simulink model "S_PIL_PVSISTEM_2026_V1"  (R2017a)
settings: Solver=VariableStepAuto  StartTime=0.0  StopTime=1.3  FixedStep=1e-6  MaxStep=1e-4  RelTol=1e-3
values from neighbouring files (symbols this model uses):
  a = 9    [M_PARAM_V1.m]    (also in M_PIL_PVSISTEM_2026_V1.m; ModTusk_V1.m)
  Alpha1 = 2*Zeta_obs*wn_obs    (= 2)    [M_PARAM_V1.m]    (also in M_PIL_PVSISTEM_2026_V1.m)
  Alpha2 = wn_obs    (= 1)    [M_PARAM_V1.m]    (also in M_PIL_PVSISTEM_2026_V1.m)
  alpha_max = 4/ts_min    (= 13333.3333333)    [M_PARAM_V1.m]    (also in M_PIL_PVSISTEM_2026_V1.m; ModTusk_V1.m)
  alpha_min = 4/ts_max    (= 259.067357513)    [M_PARAM_V1.m]    (also in M_PIL_PVSISTEM_2026_V1.m = 133.333333333; ModTusk_V1.m = 133.333333333)
  Cdc = Cdc    (= 0.0033)    [M_PARAM_V1.m]    (also in M_PIL_PVSISTEM_2026_V1.m = 0.00047)
  Cpv = Cpv    (= 0.0001)    [M_PARAM_V1.m]    (also in M_PIL_PVSISTEM_2026_V1.m = 0.0002)
  dIL = (vpv/L)*d*Ts    (= 0.46035072)    [M_PIL_PVSISTEM_2026_V1.m]
  Epsilon = Ep_cont/Ts1    [M_PARAM_V1.m]    (also in M_PIL_PVSISTEM_2026_V1.m)
  ESRCdc = ESRCdc    (= 0.2)    [M_PARAM_V1.m]    (also in M_PIL_PVSISTEM_2026_V1.m)
  ESRCpv = ESRCpv    (= 0.2)    [M_PARAM_V1.m]    (also in M_PIL_PVSISTEM_2026_V1.m)
  Fred = fs    (= 60)    [M_PARAM_V1.m]    (also in M_PIL_PVSISTEM_2026_V1.m)
  fs = 60    [M_PARAM_V1.m]    (also in M_PIL_PVSISTEM_2026_V1.m)
  Icc_calc = In/(5/100)    [M_PARAM_V1.m]    (also in M_PIL_PVSISTEM_2026_V1.m)
  K1 = Kt_acker_d    [M_PARAM_V1.m]    (also in M_PIL_PVSISTEM_2026_V1.m)
  K1y2md = Kmd(1:end-1)    [M_PARAM_V1.m]    (also in M_PIL_PVSISTEM_2026_V1.m)
  Kdpwm = 1/Ucmax    (= 0.000111111111111)    [M_PARAM_V1.m]    (also in M_PIL_PVSISTEM_2026_V1.m = 1.52590218967e-05)
  KI1 = Kp1/Ti1*Ts1    (= 760)    [M_PARAM_V1.m]    (also in M_PIL_PVSISTEM_2026_V1.m = 14.4)
  KI2 = Ki2*Ts4    [M_PARAM_V1.m]    (also in M_PIL_PVSISTEM_2026_V1.m)
  KI4 = Ki4*Ts4    [M_PARAM_V1.m]    (also in M_PIL_PVSISTEM_2026_V1.m)
  KI5 = Ki5*Ts_inv    (= 0.17765287922)    [M_PARAM_V1.m]    (also in M_PIL_PVSISTEM_2026_V1.m = 0.0710611516878)
  Kimd = -Kmd(end)    [M_PARAM_V1.m]    (also in M_PIL_PVSISTEM_2026_V1.m)
  KP1 = Kp1-KI1/2    (= 5320)    [M_PARAM_V1.m]    (also in M_PIL_PVSISTEM_2026_V1.m = 2392.8)
  KP2 = Kp2-KI2/2    [M_PARAM_V1.m]    (also in M_PIL_PVSISTEM_2026_V1.m)
  KP4 = Kp4-KI4/2    [M_PARAM_V1.m]    (also in M_PIL_PVSISTEM_2026_V1.m)
  KP5 = Kp5*Ts_inv-KI5/2    (= -0.0874937760062)    [M_PARAM_V1.m]    (also in M_PIL_PVSISTEM_2026_V1.m = -0.0349975104025)
  L = L    (= 0.0044)    [M_PARAM_V1.m]    (also in M_PIL_PVSISTEM_2026_V1.m = 0.1)
  Linv = 0.03    [M_PARAM_V1.m]    (also in M_PIL_PVSISTEM_2026_V1.m = 0.035)
  Rinv = 0.0417    [M_PARAM_V1.m]    (also in M_PIL_PVSISTEM_2026_V1.m)
  RL = RL    (= 0.494)    [M_PARAM_V1.m]    (also in M_PIL_PVSISTEM_2026_V1.m = 0.3)
  S = 10e3*3/2    (= 15000)    [M_PARAM_V1.m]    (also in M_PIL_PVSISTEM_2026_V1.m)
  Ts = Ts1    (= 0.0002)    [M_PARAM_V1.m]    (also in M_PIL_PVSISTEM_2026_V1.m)
  Ts1 = 1/Fs    (= 0.0002)    [M_PARAM_V1.m]    (also in M_PIL_PVSISTEM_2026_V1.m)
  Ts4 = 1/(4*Fc)    (= 0.000125)    [M_PARAM_V1.m]    (also in M_PIL_PVSISTEM_2026_V1.m = 5e-05)
  Ts_inv = 1/(100*Fc)    (= 5e-06)    [M_PARAM_V1.m]    (also in M_PIL_PVSISTEM_2026_V1.m = 2e-06)
  Ucmax = 9000    [M_PARAM_V1.m]    (also in M_PIL_PVSISTEM_2026_V1.m = 65535)
  vdc = 12    [M_PARAM_V1.m]    (also in M_PIL_PVSISTEM_2026_V1.m = 1000)
  vdc_ref = vdc    (= 12)    [M_PARAM_V1.m]    (also in M_PIL_PVSISTEM_2026_V1.m = 1000)
  Vf = VL/sqrt(3)    [M_PARAM_V1.m]    (also in M_PIL_PVSISTEM_2026_V1.m)
  VL = (381.051/2)    (= 190.5255)    [M_PARAM_V1.m]    (also in M_PIL_PVSISTEM_2026_V1.m)
undefined symbols (not defined in the file or in its folder): DiscIntNeverNeededParam
undefined symbols (not defined in the file): Fs
libraries: powerlib x15, powerlib_meascontrol x12, dsparch4 x3, re_lib x1
(part 1 of 2)
settings Model: ExtModeTrigDuration=10  Creator=dricl  LastModifiedBy=dricl
settings SolverCC: MaxConsecutiveZCs=100000
settings OptimizationCC: PassReuseOutputArgsAs=Individual arguments  MaxStackSize=2560
settings DebuggingCC: ParameterTunabilityLossMsg=error
settings HardwareCC: ProdBitPerPointer=32  ProdBitPerSizeT=32  ProdBitPerPtrDiffT=32  ProdLargestAtomicInteger=Long  ProdLargestAtomicFloat=Double  ProdWordSize=32  ProdLongLongMode=on  ProdHWDeviceType=ARM Compatible->ARM Cortex
settings SFSimCC: MATLABDynamicMemAlloc=off
settings RTWCC: SystemTargetFile=ert.tlc  HardwareBoard=TI Concerto F28M35x (ARM Cortex-M3)  TLCOptions=-aInlineSetEventsForThisBaseRateFcn=TLC_FALSE -aSuppressMultiTaskScheduler=TLC_FALSE -aRateBasedStepFcn=1  TemplateMakefile=ert_default_tmf  Description=Embedded Coder  GenerateReport=on  Toolchain=Texas Instruments Code Composer Studio v6 (ARM)  IncludeHyperlinkInReport=on  LaunchReport=on  CreateSILPILBlock=PIL  GenerateTraceInfo=on  GenerateTraceReport=on  GenerateTraceReportSl=on  GenerateTraceReportSf=on  GenerateTraceReportEml=on
settings CodeAppCC: ForceParamTrailComments=on  IgnoreCustomStorageClasses=off  OperatorAnnotations=on  SimulinkDataObjDesc=on  SFDataObjDesc=on  MATLABFcnDesc=on  InsertBlockDesc=on  MATLABSourceComments=on
settings ERTTargetCC: SupportVariableSizeSignals=on

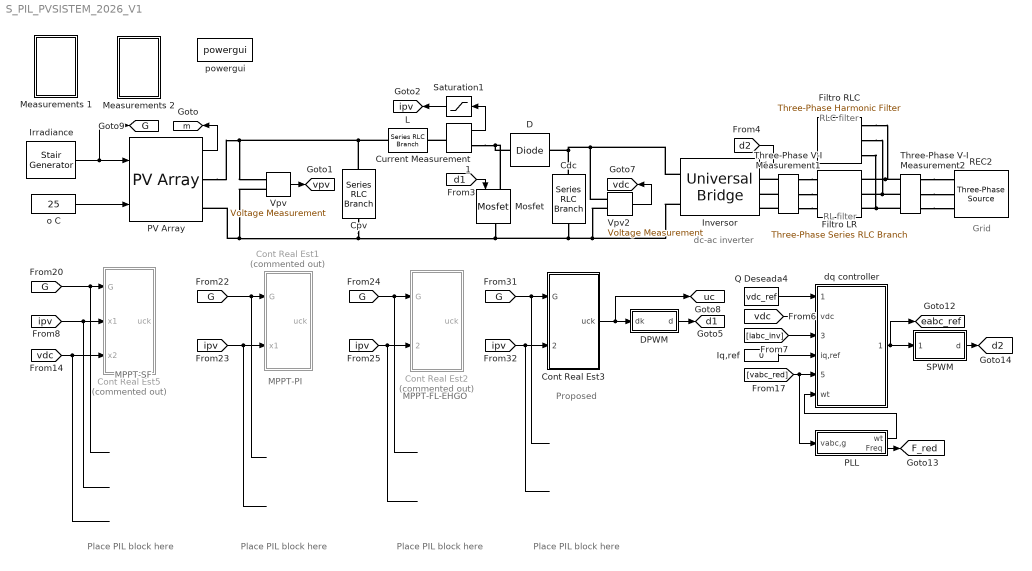
== system S_PIL_PVSISTEM_2026_V1 ==
  note: Place PIL block here
  note: Grid
  note: RLC filter
  note: MPPT-SF
  note: MPPT-PI
  note: MPPT-FL-EHGO
  note: RL filter
  note: dc-ac inverter
  note: Proposed
  note: Place PIL block here
  note: Place PIL block here
  note: Place PIL block here
  Cdc : powerlib/Elements/Series RLC Branch  LConnTagsString=__new0  RConnTagsString=__new0  BranchType=C  Resistance=ESRCdc  Inductance=1e-3  SetiL0=off  InitialCurrent=0  Capacitance=Cdc  Setx0=on  InitialVoltage=vdc_ref  Measurements=None
  Cont Real Est1 : Subsystem  Priority=7  Commented=on
  Cont Real Est2 : Subsystem  Priority=7  Commented=on
  Cont Real Est3 : Subsystem  Priority=7
  Cont Real Est5 : Subsystem  Priority=9  Commented=on
  Cpv : powerlib/Elements/Series RLC Branch  LConnTagsString=__new0  RConnTagsString=__new0  BranchType=C  Resistance=ESRCpv  Inductance=1e-3  SetiL0=off  InitialCurrent=0  Capacitance=Cpv  Setx0=on  InitialVoltage=640.8  Measurements=None
  Current Measurement1 : powerlib/Measurements/Current Measurement  PhasorSimulation=off  OutputType=Complex  PSBequivalent=0
  D : powerlib/Power Electronics/Diode  Ron=Rondiode  Lon=0  Vf=Vfdiode  IC=0  UseSnubber=0  Rs=500  Cs=250e-9  Measurements=off
  DPWM : Subsystem  AncestorBlock=plecslib_extras2/Modulators/Symmetrical PWM  mask(Symmetrical PWM){sampling=Natural (carrier starts with 0), fc=Fs, offset=0, input_limits=[0 Ucmax], output_values=[0 1]}
      mask prompts: fc "Carrier frequency (Hz):"; offset "Carrier offset (p.u.):"; input_limits "Input limits [min max]:"; output_values "Output values [off on]:"
      mask help: PWM generator with a symmetrical triangular carrier. If the input is a vector, the output is also a vector of the same width.
      mask init:
      | if numel(fc)>1 || fc<=0,
      |   error('Carrier frequency must be a positive scalar.');
      | end
      | if numel(offset)>1 || offset<0 || offset>=1,
      |   error('Carrier offset must be a scalar in the range [0; 1/fc[.');
      | end
      | if sampling == 1,
      |   offset = mod(offset+.75, 1);
      | end
      | 
      | si = [.5 mod(offset, .5)]/fc;
      mask Help: eval('plecs(''help'', ''symmetricalpwm.html'')')
      mask TypeOptions sampling: Natural (carrier starts with 0) | Natural (carrier starts with 1) | Regular (double edge) | Regular (single edge)
  Filtro LR : powerlib/Elements/Three-Phase Series RLC Branch  LConnTagsString=A|B|C  RConnTagsString=A|B|C  BranchType=RL  Resistance=Rinv  Inductance=Linv  Capacitance=1e-6  Measurements=None
  Filtro RLC : powerlib/Elements/Three-Phase Harmonic Filter  LConnTagsString=A|B|C  FilterType=Single-tuned  FilterConnection=Y (grounded)  ParNom=[VL fs]  Qc=S*0.001  Fr=[31.42*60]  Frd=[40*fs 80*fs]  Q=5  Measurements=None
      settings: AttributesFormatString=\n  SourceProductName=Simscape Power Systems  SourceProductBaseCode=PS
  Inversor : powerlib/Power Electronics/Universal Bridge  Arms=3  SnubberResistance=1e5  SnubberCapacitance=inf  Device=IGBT / Diodes  Ron=1e-3  Lon=0  ForwardVoltages="[  0  0  ]"  ForwardVoltage=0  GTOparameters=[ 10e-6 , 20e-6 ]  IGBTparameters=[ 1e-6 , 2e-6 ]  Measurements=None  Measurements_2=None  converterType=Rectifier
  Iq,ref : Constant  Value=0  SampleTime=Ts4
  Irradiance : powerlib_meascontrol/Pulse & Signal Generators/Stair Generator  t=[0, 0.1, 0.3, 0.5, 0.7, 0.9, 1.1]  e=[0, 1000, 400, 800, 500, 900, 600]  Ts=0
      settings: SourceProductName=Simscape Power Systems
  L : powerlib/Elements/Series RLC Branch  LConnTagsString=__new0  RConnTagsString=__new0  BranchType=L  Resistance=RL  Inductance=L  SetiL0=off  InitialCurrent=0  Capacitance=1e-6  Setx0=off  InitialVoltage=0  Measurements=None
  Measurements 1 : Subsystem
  Measurements 2 : Subsystem
  Mosfet : powerlib/Power Electronics/Mosfet  Ron=Ronfet  Lon=0  Rd=0  Vfd=0  IC=0  Rs=1e5  Cs=inf  Measurements=off
  PLL : Subsystem
  PV Array : re_lib/Solar/PV Array  Npar=No_Cadenas_Paralelo  Nser=No_Modulos_PorCadena  PlotType=array @ 25 deg.C & specified irradiances  S_vec=[1037]  Temp_C_vec="[ 45 25  0]"  ModuleName=Canadian Solar CS6X-280P  PlotWhenSelected=off  Pm=279.816  Ncell=72  Voc=44.2  Isc=8.42  Vm=35.6  Im=7.86  beta_Voc_pc=-0.39  alpha_Isc_pc=0.06  beta_Voc=-0.17238  alpha_Isc=0.005052  IL=8.4417  I0=7.7188e-10  nI=1.0345  Rsh=300.2269  Rs=0.38773  BAL=off  Tc=1e-6  Tfilter=5e-5
  Q Deseada4 : Constant  Value=vdc_ref  SampleTime=Ts4
  REC2 : powerlib/Electrical Sources/Three-Phase Source  InternalConnection=Yg  VoltagePhases=on  Voltage=VL  PhaseAngle=0  Voltage_phases=[VL/sqrt(3) VL/sqrt(3) VL/sqrt(3)]  PhaseAngles_phases=[0 -120 +120]  Frequency=Fred  NonIdealSource=on  SpecifyImpedance=on  Resistance=25e3^2/10e6/5  Inductance=25e3^2/10e6/377  ShortCircuitLevel=Icc_calc*2  BaseVoltage=VL  XRratio=7  BusType=swing  Pref=-500e3  Qref=0  Prefabc=[10e3, 10e3, 10e3]  Qrefabc=[0, 0, 0]  Qmin=-inf  Qmax=inf
  SPWM : Subsystem
  Saturation1 : Saturate  UpperLimit=inf  LowerLimit=0
  Three-Phase V-I Measurement1 : powerlib/Measurements/Three-Phase V-I Measurement  VoltageMeasurement=phase-to-ground  SetLabelV=on  LabelV=vabc_inv  Vpu=off  VpuLL=off  CurrentMeasurement=yes  SetLabelI=on  LabelI=iabc_inv  Ipu=off  Pbase=100e6  Vbase=500e3  OutputType=Complex  PhasorSimulation=off  PSBequivalent=0
  Three-Phase V-I Measurement2 : powerlib/Measurements/Three-Phase V-I Measurement  VoltageMeasurement=phase-to-ground  SetLabelV=on  LabelV=vabc_red  Vpu=off  VpuLL=off  CurrentMeasurement=yes  SetLabelI=on  LabelI=iabc_red  Ipu=off  Pbase=100e6  Vbase=500e3  OutputType=Complex  PhasorSimulation=off  PSBequivalent=0
  Vpv : powerlib/Measurements/Voltage Measurement  PhasorSimulation=off  OutputType=Complex  PSBequivalent=0
  Vpv2 : powerlib/Measurements/Voltage Measurement  PhasorSimulation=off  OutputType=Complex  PSBequivalent=0
  dq controller : Subsystem
  o C : Constant  Value=25
  powergui : powerlib/powergui  Priority=1  SimulationMode=Continuous  SampleTime=1e-6  frequency=60  Iterations=50  frequencyindice=0  Pbase=100e6  ErrMax=1e-4  UnitsV=kV  UnitsW=MW  buscounter=0  FunctionMessages=off  echomessages=off  EnableUseOfTLC=off  CurrentSourceSwitches=off  DisableSnubberDevices=off  DisableRonSwitches=off  DisableVfSwitches=off  DisplayEquations=off  SolverType=Tustin/Backward Euler (TBE)  Interpol=off  ExternalGateDelay=off  methode=off  Ts=100  x0status=blocks  SPID=on  SwTol=0  HookPort=off  RestoreLinks=warning  ResistiveCurrentMeasurement=off  Frange=[0:2:500]  Ylog=off  Xlog=on  ShowGrid=off  save=off  variable=ZData  structure=logsout  ZoomFFT=off  StartTime=1.25  cycles=3  DisplayStyle=1  fundamental=60  FreqAxis=off  MaxFrequency=1000  frequencyindicesteady=1  RmsSteady=1  display=off
  tag scope: F_red=global, G=global, d1=global, d2=global, eabc_ref=global, ipv=global, m=global, uc=global, vdc=global, vpv=global
  wires:
  [iabc_inv] -> dq controller/3(iabc,inv)
  Iq,ref/1 -> dq controller/4(iq,ref)
  Vpv2/1 -> [vdc]
  PLL/2(Freq) -> [F_red]
  SPWM/1(d) -> [d2]
  DPWM/1(d) -> [d1]
  o C/1 -> PV Array/2
  PLL/1(wt) -> dq controller/6(wt)
  [vabc_red] -> dq controller/5(vabc,red), PLL/1(vabc,g)
  [d2] -> Inversor/1
  Vpv/1 -> [vpv]
  dq controller/1(eabc,ref) -> [eabc_ref], SPWM/1(eabc,ref)
  [d1] -> Mosfet/1
  PV Array/1 -> [m]
  [ipv] -> Cont Real Est1/2(x1)
  [ipv] -> Cont Real Est2/2(x1 = ipv)
  [ipv] -> Cont Real Est5/2(x1)
  [G] -> Cont Real Est5/1(G)
  [G] -> Cont Real Est2/1(G)
  [G] -> Cont Real Est3/1(G)
  Q Deseada4/1 -> dq controller/1(vdc,ref)
  [vdc] -> dq controller/2(vdc)
  Irradiance/1 -> [G], PV Array/1
  Saturation1/1 -> [ipv]
  Current Measurement1/1 -> Saturation1/1
  [ipv] -> Cont Real Est3/2(x1 = ipv)
  [vdc] -> Cont Real Est5/3(x2)
  [G] -> Cont Real Est1/1(G)
  Cont Real Est3/1(uck) -> [uc], DPWM/1(dk)
  connections:
  PV Array/RConn1 -- Vpv/LConn1 -- Cpv/LConn1 -- L/LConn1
  Filtro RLC/LConn1 -- Filtro LR/RConn1 -- Three-Phase V-I Measurement2/LConn1
  Three-Phase V-I Measurement2/RConn1 -- REC2/RConn1
  Cdc/RConn1 -- Vpv2/LConn2 -- Inversor/RConn2 -- Cpv/RConn1 -- Vpv/LConn2 -- PV Array/RConn2 -- Mosfet/RConn1
  Filtro RLC/LConn2 -- Filtro LR/RConn2 -- Three-Phase V-I Measurement2/LConn2
  Three-Phase V-I Measurement2/RConn2 -- REC2/RConn2
  D/RConn1 -- Vpv2/LConn1 -- Inversor/RConn1 -- Cdc/LConn1
  Filtro RLC/LConn3 -- Filtro LR/RConn3 -- Three-Phase V-I Measurement2/LConn3
  Three-Phase V-I Measurement2/RConn3 -- REC2/RConn3
  D/LConn1 -- Current Measurement1/RConn1 -- Mosfet/LConn1
  Three-Phase V-I Measurement1/RConn1 -- Filtro LR/LConn1
  Three-Phase V-I Measurement1/RConn2 -- Filtro LR/LConn2
  Three-Phase V-I Measurement1/RConn3 -- Filtro LR/LConn3
  Three-Phase V-I Measurement1/LConn2 -- Inversor/LConn2
  Current Measurement1/LConn1 -- L/RConn1
  Three-Phase V-I Measurement1/LConn1 -- Inversor/LConn1
  Three-Phase V-I Measurement1/LConn3 -- Inversor/LConn3

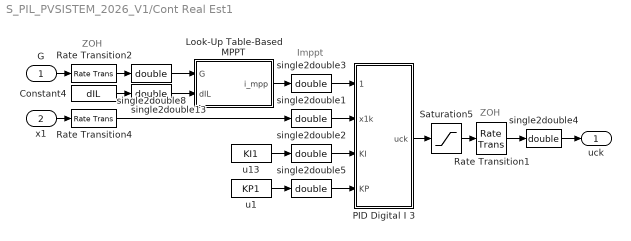
== system S_PIL_PVSISTEM_2026_V1/Cont Real Est1 ==
  note: Imppt
  note: ZOH
  note: ZOH
  G : Inport
  x1 : Inport  Port=2
  Constant4 : Constant  Value=dIL  SampleTime=Ts1
  Look-Up Table-Based MPPT : MATLAB Function  TreatAsAtomicUnit=on
  PID Digital I 3 : MATLAB Function  TreatAsAtomicUnit=on
  Rate Transition1 : RateTransition  Deterministic=off  OutPortSampleTime=Ts1
  Rate Transition2 : RateTransition  Deterministic=off  OutPortSampleTime=Ts1
  Rate Transition4 : RateTransition  Deterministic=off  OutPortSampleTime=Ts1
  Saturation5 : Saturate  UpperLimit=Ucmax  LowerLimit=0
  single2double{1..5,8,13} (7 alike) : DataTypeConversion  OutDataTypeStr=double
  u1 : Constant  Value=KP1  SampleTime=Ts1
  u13 : Constant  Value=KI1  SampleTime=Ts1
  uck : Outport
  wires:
  u1/1 -> single2double5/1
  u13/1 -> single2double2/1
  PID Digital I 3/1(uck) -> Saturation5/1
  single2double3/1 -> PID Digital I 3/1(x1k_ref)
  single2double1/1 -> PID Digital I 3/2(x1k)
  single2double4/1 -> uck/1
  single2double2/1 -> PID Digital I 3/3(KI)
  single2double5/1 -> PID Digital I 3/4(KP)
  single2double13/1 -> Look-Up Table-Based MPPT/2(dIL)
  Constant4/1 -> single2double13/1
  Look-Up Table-Based MPPT/1(i_mpp) -> single2double3/1
  single2double8/1 -> Look-Up Table-Based MPPT/1(G)
  G/1 -> Rate Transition2/1
  Rate Transition2/1 -> single2double8/1
  x1/1 -> Rate Transition4/1
  Rate Transition4/1 -> single2double1/1
  Saturation5/1 -> Rate Transition1/1
  Rate Transition1/1 -> single2double4/1

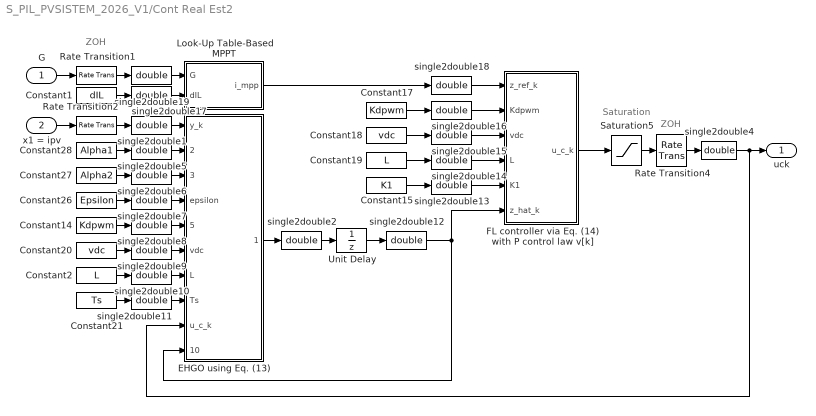
== system S_PIL_PVSISTEM_2026_V1/Cont Real Est2 ==
  note: Saturation
  note: ZOH
  note: ZOH
  G : Inport
  x1 = ipv : Inport  Port=2
  Constant1 : Constant  Value=dIL  SampleTime=Ts1
  Constant14 : Constant  Value=Kdpwm  SampleTime=Ts1
  Constant15 : Constant  Value=K1  SampleTime=Ts1
  Constant17 : Constant  Value=Kdpwm  SampleTime=Ts1
  Constant18 : Constant  Value=vdc  SampleTime=Ts1
  Constant19 : Constant  Value=L  SampleTime=Ts1
  Constant2 : Constant  Value=L  SampleTime=Ts1
  Constant20 : Constant  Value=vdc  SampleTime=Ts1
  Constant21 : Constant  Value=Ts  SampleTime=Ts1
  Constant26 : Constant  Value=Epsilon  SampleTime=Ts1
  Constant27 : Constant  Value=Alpha2  SampleTime=Ts1
  Constant28 : Constant  Value=Alpha1  SampleTime=Ts1
  EHGO using Eq. (13) : MATLAB Function  TreatAsAtomicUnit=on
  FL controller via Eq. (14) with P control law v[k] : MATLAB Function  TreatAsAtomicUnit=on
  Look-Up Table-Based MPPT : MATLAB Function  TreatAsAtomicUnit=on
  Rate Transition1 : RateTransition  Deterministic=off  OutPortSampleTime=Ts1
  Rate Transition2 : RateTransition  Deterministic=off  OutPortSampleTime=Ts1
  Rate Transition4 : RateTransition  Deterministic=off  OutPortSampleTime=Ts1
  Saturation5 : Saturate  UpperLimit=Ucmax  LowerLimit=0
  Unit Delay : UnitDelay  SampleTime=Ts1
  single2double{1..2,4..19} (18 alike) : DataTypeConversion  OutDataTypeStr=double
  uck : Outport
  wires:
  FL controller via Eq. (14) with P control law v[k]/1(u_c_k) -> Saturation5/1
  single2double18/1 -> FL controller via Eq. (14) with P control law v[k]/1(z_ref_k)
  single2double1/1 -> EHGO using Eq. (13)/1(y_k)
  single2double4/1 -> EHGO using Eq. (13)/9(u_c_k), uck/1
  Constant28/1 -> single2double5/1
  single2double5/1 -> EHGO using Eq. (13)/2(alpha_1)
  Constant27/1 -> single2double6/1
  single2double6/1 -> EHGO using Eq. (13)/3(alpha_2)
  Constant26/1 -> single2double7/1
  single2double7/1 -> EHGO using Eq. (13)/4(epsilon)
  Constant14/1 -> single2double8/1
  single2double8/1 -> EHGO using Eq. (13)/5(Kdpwm)
  Constant20/1 -> single2double9/1
  single2double9/1 -> EHGO using Eq. (13)/6(vdc)
  Constant2/1 -> single2double10/1
  single2double10/1 -> EHGO using Eq. (13)/7(L)
  Constant21/1 -> single2double11/1
  single2double11/1 -> EHGO using Eq. (13)/8(Ts)
  Unit Delay/1 -> single2double12/1
  single2double12/1 -> FL controller via Eq. (14) with P control law v[k]/6(z_hat_k), EHGO using Eq. (13)/10(z_hat_k)
  Constant15/1 -> single2double13/1
  Constant19/1 -> single2double14/1
  Constant18/1 -> single2double15/1
  Constant17/1 -> single2double16/1
  single2double16/1 -> FL controller via Eq. (14) with P control law v[k]/2(Kdpwm)
  single2double15/1 -> FL controller via Eq. (14) with P control law v[k]/3(vdc)
  single2double14/1 -> FL controller via Eq. (14) with P control law v[k]/4(L)
  single2double13/1 -> FL controller via Eq. (14) with P control law v[k]/5(K1)
  EHGO using Eq. (13)/1(z_hat_next) -> single2double2/1
  single2double2/1 -> Unit Delay/1
  Constant1/1 -> single2double17/1
  single2double17/1 -> Look-Up Table-Based MPPT/2(dIL)
  single2double19/1 -> Look-Up Table-Based MPPT/1(G)
  G/1 -> Rate Transition1/1
  x1 = ipv/1 -> Rate Transition2/1
  Rate Transition1/1 -> single2double19/1
  Rate Transition2/1 -> single2double1/1
  Saturation5/1 -> Rate Transition4/1
  Rate Transition4/1 -> single2double4/1
  Look-Up Table-Based MPPT/1(i_mpp) -> single2double18/1

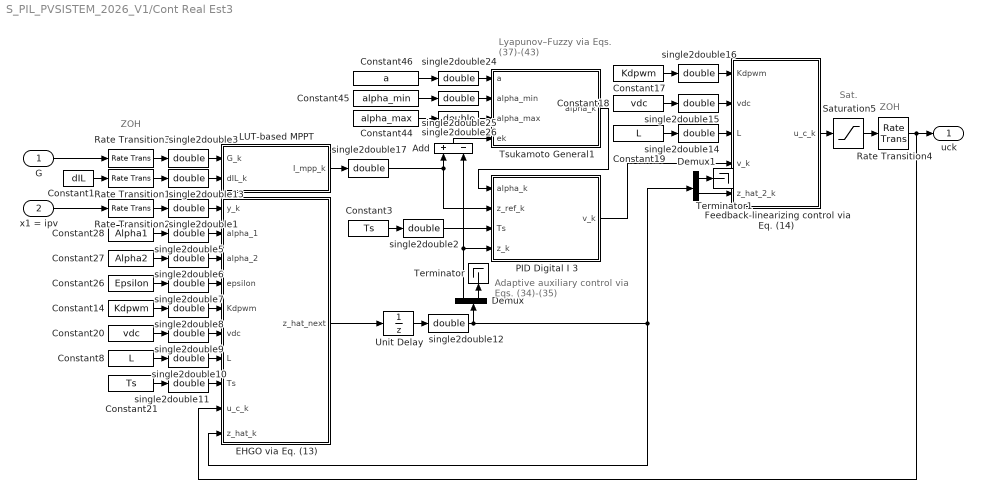
== system S_PIL_PVSISTEM_2026_V1/Cont Real Est3 ==
  note: Adaptive auxiliary
      | control via
      | Eqs. (34)-(35)
  note: Lyapunov–Fuzzy
      | via Eqs. (37)-(43)
  note: ZOH
  note: Sat.
  note: ZOH
  G : Inport
  x1 = ipv : Inport  Port=2
  Add : Sum  Inputs=+-
  Constant1 : Constant  Value=dIL  SampleTime=Ts1
  Constant14 : Constant  Value=Kdpwm  SampleTime=Ts1
  Constant17 : Constant  Value=Kdpwm  SampleTime=Ts1
  Constant18 : Constant  Value=vdc  SampleTime=Ts1
  Constant19 : Constant  Value=L  SampleTime=Ts1
  Constant20 : Constant  Value=vdc  SampleTime=Ts1
  Constant21 : Constant  Value=Ts  SampleTime=Ts1
  Constant26 : Constant  Value=Epsilon  SampleTime=Ts1
  Constant27 : Constant  Value=Alpha2  SampleTime=Ts1
  Constant28 : Constant  Value=Alpha1  SampleTime=Ts1
  Constant3 : Constant  Value=Ts  SampleTime=Ts1
  Constant44 : Constant  Value=alpha_max  SampleTime=Ts1
  Constant45 : Constant  Value=alpha_min  SampleTime=Ts1
  Constant46 : Constant  Value=a  SampleTime=Ts1
  Constant8 : Constant  Value=L  SampleTime=Ts1
  Demux : Demux  Outputs=2
  Demux1 : Demux  Outputs=2
  EHGO via Eq. (13) : MATLAB Function  TreatAsAtomicUnit=on
  Feedback-linearizing control via Eq. (14) : MATLAB Function  TreatAsAtomicUnit=on
  LUT-based MPPT : MATLAB Function  TreatAsAtomicUnit=on
  PID Digital I 3 : MATLAB Function  TreatAsAtomicUnit=on
  Rate Transition{1..4} (4 alike) : RateTransition  Deterministic=off  OutPortSampleTime=Ts1
  Saturation5 : Saturate  UpperLimit=Ucmax  LowerLimit=0
  Terminator : Terminator
  Terminator1 : Terminator
  Tsukamoto General1 : MATLAB Function  TreatAsAtomicUnit=on
  Unit Delay : UnitDelay  SampleTime=Ts1
  single2double{1..3,5..17,24..26} (19 alike) : DataTypeConversion  OutDataTypeStr=double
  uck : Outport
  wires:
  Feedback-linearizing control via Eq. (14)/1(u_c_k) -> Saturation5/1
  single2double1/1 -> EHGO via Eq. (13)/1(y_k)
  Rate Transition4/1 -> uck/1, EHGO via Eq. (13)/9(u_c_k)
  Constant28/1 -> single2double5/1
  single2double5/1 -> EHGO via Eq. (13)/2(alpha_1)
  Constant27/1 -> single2double6/1
  single2double6/1 -> EHGO via Eq. (13)/3(alpha_2)
  Constant26/1 -> single2double7/1
  single2double7/1 -> EHGO via Eq. (13)/4(epsilon)
  Constant14/1 -> single2double8/1
  single2double8/1 -> EHGO via Eq. (13)/5(Kdpwm)
  Constant20/1 -> single2double9/1
  single2double9/1 -> EHGO via Eq. (13)/6(vdc)
  Constant8/1 -> single2double10/1
  single2double10/1 -> EHGO via Eq. (13)/7(L)
  Constant21/1 -> single2double11/1
  single2double11/1 -> EHGO via Eq. (13)/8(Ts)
  Unit Delay/1 -> single2double12/1
  single2double12/1 -> Demux/1, Demux1/1, EHGO via Eq. (13)/10(z_hat_k)
  Constant19/1 -> single2double14/1
  Constant18/1 -> single2double15/1
  Constant17/1 -> single2double16/1
  single2double16/1 -> Feedback-linearizing control via Eq. (14)/1(Kdpwm)
  single2double15/1 -> Feedback-linearizing control via Eq. (14)/2(vdc)
  single2double14/1 -> Feedback-linearizing control via Eq. (14)/3(L)
  EHGO via Eq. (13)/1(z_hat_next) -> Unit Delay/1
  Constant3/1 -> single2double2/1
  single2double2/1 -> PID Digital I 3/3(Ts)
  Constant46/1 -> single2double24/1
  single2double25/1 -> Tsukamoto General1/2(alpha_min)
  Constant44/1 -> single2double26/1
  single2double26/1 -> Tsukamoto General1/3(alpha_max)
  single2double24/1 -> Tsukamoto General1/1(a)
  Constant45/1 -> single2double25/1
  Add/1 -> Tsukamoto General1/4(ek)
  LUT-based MPPT/1(I_mpp_k) -> single2double17/1
  Demux/2 -> Terminator/1
  Demux/1 -> PID Digital I 3/4(z_k), Add/2
  Tsukamoto General1/1(alpha_k) -> PID Digital I 3/1(alpha_k)
  single2double3/1 -> LUT-based MPPT/1(G_k)
  single2double13/1 -> LUT-based MPPT/2(dIL_k)
  Demux1/2 -> Feedback-linearizing control via Eq. (14)/5(z_hat_2_k)
  Demux1/1 -> Terminator1/1
  PID Digital I 3/1(v_k) -> Feedback-linearizing control via Eq. (14)/4(v_k)
  single2double17/1 -> PID Digital I 3/2(z_ref_k), Add/1
  G/1 -> Rate Transition3/1
  x1 = ipv/1 -> Rate Transition2/1
  Rate Transition2/1 -> single2double1/1
  Rate Transition3/1 -> single2double3/1
  Saturation5/1 -> Rate Transition4/1
  Constant1/1 -> Rate Transition1/1
  Rate Transition1/1 -> single2double13/1

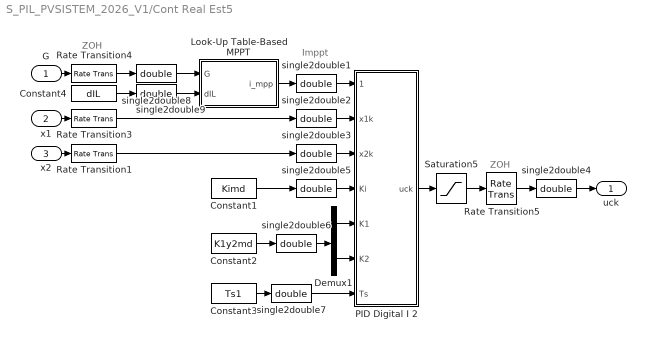
== system S_PIL_PVSISTEM_2026_V1/Cont Real Est5 ==
  note: Imppt
  note: ZOH
  note: ZOH
  G : Inport
  x1 : Inport  Port=2
  x2 : Inport  Port=3
  Constant1 : Constant  Value=Kimd  SampleTime=Ts1
  Constant2 : Constant  Value=K1y2md  SampleTime=Ts1
  Constant3 : Constant  Value=Ts1  SampleTime=Ts1
  Constant4 : Constant  Value=dIL  SampleTime=Ts1
  Demux1 : Demux  Outputs=2
  Look-Up Table-Based MPPT : MATLAB Function  TreatAsAtomicUnit=on
  PID Digital I 2 : MATLAB Function  TreatAsAtomicUnit=on
  Rate Transition{1,3..5} (4 alike) : RateTransition  Deterministic=off  OutPortSampleTime=Ts1
  Saturation5 : Saturate  UpperLimit=Ucmax  LowerLimit=0
  single2double{1..9} (9 alike) : DataTypeConversion  OutDataTypeStr=double
  uck : Outport
  wires:
  PID Digital I 2/1(uck) -> Saturation5/1
  Constant1/1 -> single2double5/1
  Demux1/1 -> PID Digital I 2/5(K1)
  single2double1/1 -> PID Digital I 2/1(x1k_Ref)
  single2double2/1 -> PID Digital I 2/2(x1k)
  single2double3/1 -> PID Digital I 2/3(x2k)
  single2double4/1 -> uck/1
  single2double5/1 -> PID Digital I 2/4(Ki)
  single2double7/1 -> PID Digital I 2/7(Ts)
  Constant4/1 -> single2double9/1
  single2double9/1 -> Look-Up Table-Based MPPT/2(dIL)
  single2double8/1 -> Look-Up Table-Based MPPT/1(G)
  Look-Up Table-Based MPPT/1(i_mpp) -> single2double1/1
  single2double6/1 -> Demux1/1
  Demux1/2 -> PID Digital I 2/6(K2)
  Constant2/1 -> single2double6/1
  Constant3/1 -> single2double7/1
  Rate Transition4/1 -> single2double8/1
  G/1 -> Rate Transition4/1
  Rate Transition3/1 -> single2double2/1
  x1/1 -> Rate Transition3/1
  x2/1 -> Rate Transition1/1
  Rate Transition1/1 -> single2double3/1
  Saturation5/1 -> Rate Transition5/1
  Rate Transition5/1 -> single2double4/1

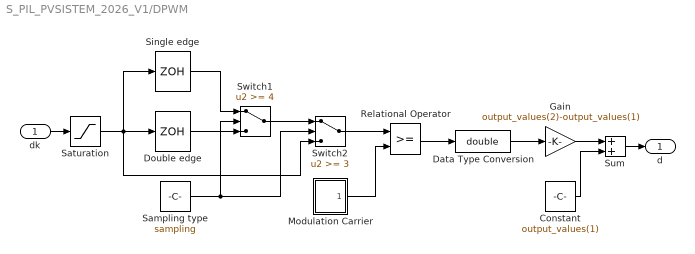
== system S_PIL_PVSISTEM_2026_V1/DPWM ==
  dk : Inport
  Constant : Constant  Value=output_values(1)
  Data Type Conversion : DataTypeConversion  OutDataTypeStr=double  SaturateOnIntegerOverflow=on  RndMeth=Zero
  Double edge : ZeroOrderHold  SampleTime=si
  Gain : Gain  Gain=output_values(2)-output_values(1)  SaturateOnIntegerOverflow=on  OutDataTypeStr=Inherit: Same as input  ParamDataTypeStr=Inherit: Same as input
  Modulation Carrier : Subsystem  mask(Symmetric Triangle Generator){fc=fc, offset=mod(offset+.5, 1), range=input_limits}
      mask prompts: fc "Carrier frequency (Hz):"; offset "Carrier offset (p.u.):"; range "Signal range [min max]:"
      mask help: Generates a symmetrical triangular signal with output values between 0 and 1. The block forces the Simulink solver to output all tips of the signal. The output can therefore be used as a carrier signal for PWM.
      mask init:
      | if numel(fc)>1 || fc<=0,
      |   error('Carrier frequency must be a positive scalar.');
      | end
      | if numel(offset)>1 || offset<0 || offset>=1,
      |   error('Carrier offset must be a scalar in the interval [0; 1[.');
      | end
      | if numel(range)~=2,
      |   error('Signal range must be a two-element vector.')
      | end
      | if range(1)>=range(2),
      |   error('Signal range must be specified as [min max].')
      | end
      | 
      | carrier_t = [0 offset mod(1/2+offset, 1) 1]/fc;
      | carrier_v0 = 1-2*abs(offset-.5);
      | carrier_v = range(1)+[carrier_v0 0 1 carrier_v0]*diff(range);
      | [carrier_t, idx] = unique(carrier_t);
      | carrier_v = carrier_v(idx);
      | si = [.5 mod(offset, .5)]/fc;
      | 
      | L = length(carrier_t);
      | disp_seq_t = repmat(carrier_t(:),1,3) + ones(L,1)*[0,1,2]/fc;
      | disp_seq_v = repmat(carrier_v(:),1,3);
      mask Display: plot(disp_seq_t, disp_seq_v)
  Relational Operator : RelationalOperator  RndMeth=Nearest  InputSameDT=on
  Sampling type : Constant  Value=sampling
  Saturation : Saturate  UpperLimit=input_limits(2)  LowerLimit=input_limits(1)
  Single edge : ZeroOrderHold  SampleTime=[1 offset]/fc
  Sum : Sum  SaturateOnIntegerOverflow=on  InputSameDT=on  OutDataTypeStr=Inherit: Same as first input
  Switch1 : Switch  Threshold=4  SaturateOnIntegerOverflow=on  InputSameDT=on
  Switch2 : Switch  Threshold=3  SaturateOnIntegerOverflow=on  InputSameDT=on
  d : Outport
  wires:
  Data Type Conversion/1 -> Gain/1
  Constant/1 -> Sum/2
  Gain/1 -> Sum/1
  Sum/1 -> d/1
  Relational Operator/1 -> Data Type Conversion/1
  Switch2/1 -> Relational Operator/1
  Sampling type/1 -> Switch1/2, Switch2/2
  Single edge/1 -> Switch1/1
  Saturation/1 -> Double edge/1, Single edge/1, Switch2/3
  dk/1 -> Saturation/1
  Modulation Carrier/1(Out) -> Relational Operator/2
  Switch1/1 -> Switch2/1
  Double edge/1 -> Switch1/3

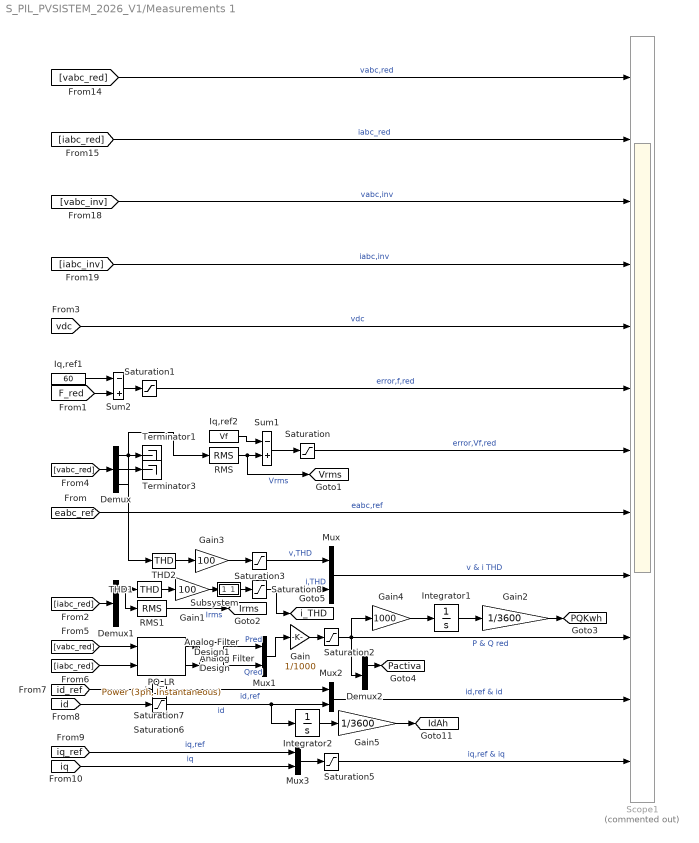
== system S_PIL_PVSISTEM_2026_V1/Measurements 1 ==
  Analog Filter Design : dsparch4/Analog Filter Design  method=Butterworth  filttype=Lowpass  N=8  Wlo=4000  Whi=80  Rp=2  Rs=40
  Analog Filter Design1 : dsparch4/Analog Filter Design  method=Butterworth  filttype=Lowpass  N=8  Wlo=4000  Whi=80  Rp=2  Rs=40
  Demux : Demux  Outputs=3
  Demux1 : Demux  Outputs=3
  Demux2 : Demux  Outputs=2
  Gain : Gain  Gain=1/1000
  Gain1 : Gain  Gain=100
  Gain2 : Gain  Gain=1/3600
  Gain3 : Gain  Gain=100
  Gain4 : Gain  Gain=1000
  Gain5 : Gain  Gain=1/3600
  Integrator1 : Integrator  ZeroCross=off
  Integrator2 : Integrator  ZeroCross=off
  Iq,ref1 : Constant  Value=60  SampleTime=Ts4
  Iq,ref2 : Constant  Value=Vf  SampleTime=Ts4
  Mux{,1..3} (4 alike) : Mux  Inputs=2
  PQ_LR : powerlib_meascontrol/Measurements/Power (3ph, Instantaneous)
      settings: SourceProductName=Simscape Power Systems
  RMS : powerlib_meascontrol/Measurements/RMS  TrueRMS=on  Freq=60  RMSInit=0  Ts=0
  RMS1 : powerlib_meascontrol/Measurements/RMS  TrueRMS=on  Freq=60  RMSInit=0  Ts=0
  Saturation : Saturate  UpperLimit=5.5  LowerLimit=-5.5
  Saturation1 : Saturate  UpperLimit=1  LowerLimit=-1
  Saturation2 : Saturate  UpperLimit=20  LowerLimit=0
  Saturation3 : Saturate  UpperLimit=20  LowerLimit=0
  Saturation5 : Saturate  UpperLimit=100  LowerLimit=0
  Saturation6 : Saturate  UpperLimit=inf  LowerLimit=0
  Saturation7 : Saturate  UpperLimit=inf  LowerLimit=0
  Saturation8 : Saturate  UpperLimit=50  LowerLimit=0
  Scope1 : Scope  Commented=on  NumInputPorts=12
  Subsystem : Subsystem
  Sum1 : Sum  Inputs=-+
  Sum2 : Sum  Inputs=-+
  THD1 : powerlib_meascontrol/Measurements/THD  Freq=60  Ts=0
  THD2 : powerlib_meascontrol/Measurements/THD  Freq=60  Ts=0
  Terminator1 : Terminator
  Terminator3 : Terminator
  tag scope: IdAh=global, Irms=global, PQKwh=global, Pactiva=global, Vrms=global, i_THD=global
  wires:
  Saturation/1 -> Scope1/7  "error,Vf,red"
  [vabc_red] -> Scope1/1  "vabc,red"
  [eabc_ref] -> Scope1/8  "eabc,ref"
  [iabc_red] -> Scope1/2  "iabc_red"
  Demux/1 -> THD2/1, RMS/1
  [vdc] -> Scope1/5  "vdc"
  [iabc_inv] -> Scope1/4  "iabc,inv"
  [vabc_inv] -> Scope1/3  "vabc,inv"
  Sum1/1 -> Saturation/1
  RMS/1 -> [Vrms], Sum1/2  "Vrms"
  Demux/2 -> Terminator3/1
  Demux/3 -> Terminator1/1
  [vabc_red] -> Demux/1
  [F_red] -> Sum2/2
  Iq,ref2/1 -> Sum1/1
  Iq,ref1/1 -> Sum2/1
  Saturation1/1 -> Scope1/6  "error,f,red"
  Sum2/1 -> Saturation1/1
  Demux1/1 -> RMS1/1, THD1/1
  THD2/1 -> Gain3/1
  THD1/1 -> Gain1/1
  Mux/1 -> Scope1/9  "v & i THD"
  [vabc_red] -> PQ_LR/1
  [iabc_red] -> PQ_LR/2
  PQ_LR/1 -> Analog Filter Design/1
  Analog Filter Design/1 -> Mux1/1  "Pred"
  PQ_LR/2 -> Analog Filter Design1/1
  Analog Filter Design1/1 -> Mux1/2  "Qred"
  Saturation2/1 -> Demux2/1, Gain4/1, Scope1/10  "P & Q red"
  Gain/1 -> Saturation2/1
  Mux1/1 -> Gain/1
  Mux3/1 -> Saturation5/1
  [iq] -> Mux3/2  "iq"
  [id] -> Saturation6/1
  [iq_ref] -> Mux3/1  "iq,ref"
  [id_ref] -> Saturation7/1
  Mux2/1 -> Scope1/11  "id,ref & id"
  Saturation5/1 -> Scope1/12  "iq,ref & iq"
  RMS1/1 -> [Irms]  "Irms"
  Saturation6/1 -> Integrator2/1, Mux2/2  "id"
  Saturation7/1 -> Mux2/1  "id,ref"
  Gain3/1 -> Saturation3/1
  Saturation3/1 -> Mux/1  "v,THD"
  Saturation8/1 -> [i_THD], Mux/2  "i,THD"
  Integrator2/1 -> Gain5/1
  Integrator1/1 -> Gain2/1
  Demux2/1 -> [Pactiva]
  Gain2/1 -> [PQKwh]
  Gain4/1 -> Integrator1/1
  Gain5/1 -> [IdAh]
  [iabc_red] -> Demux1/1
  Gain1/1 -> Subsystem/1(I)
  Subsystem/1(O) -> Saturation8/1

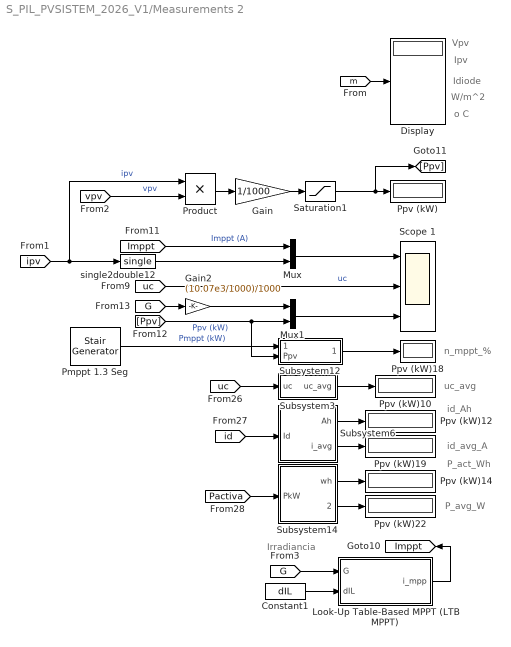
== system S_PIL_PVSISTEM_2026_V1/Measurements 2 ==
  note: W/m^2
  note: Idiode
  note: Vpv
  note: Ipv
  note: o C
  note: Irradiancia
  note: P_act_Wh
  note: n_mppt_%
  note: id_avg_A
  note: id_Ah
  note: uc_avg
  note: P_avg_W
  Constant1 : Constant  Value=dIL  SampleTime=Ts1
  Display : Display
  Gain : Gain  Gain=1/1000
  Gain2 : Gain  Gain=(10.07e3/1000)/1000
  Look-Up Table-Based MPPT (LTB MPPT) : MATLAB Function  TreatAsAtomicUnit=on
  Mux : Mux  Inputs=2
  Mux1 : Mux  Inputs=2
  Pmppt 1.3 Seg : powerlib_meascontrol/Pulse & Signal Generators/Stair Generator  t=[0, 0.1, 0.3, 0.5, 0.7, 0.9, 1.1]  e=[0, 10.07, 4.040, 8.099, 5.066, 9.090, 6.086]*0.99755  Ts=0
      settings: SourceProductName=Simscape Power Systems
  Ppv (kW){,10,12,14,18..19,22} (7 alike) : Display
  Product : Product
  Saturation1 : Saturate  UpperLimit=inf  LowerLimit=0
  Scope 1 : Scope  NumInputPorts=3
  Subsystem12 : Subsystem
  Subsystem14 : Subsystem
  Subsystem3 : Subsystem
  Subsystem6 : Subsystem
  single2double12 : DataTypeConversion  OutDataTypeStr=single
  tag scope: Imppt=global
  wires:
  [m] -> Display/1
  Constant1/1 -> Look-Up Table-Based MPPT (LTB MPPT)/2(dIL)
  Look-Up Table-Based MPPT (LTB MPPT)/1(i_mpp) -> [Imppt]
  [G] -> Look-Up Table-Based MPPT (LTB MPPT)/1(G)
  Subsystem3/1(uc_avg) -> Ppv (kW)10/1
  [Ppv] -> Mux1/2, Subsystem12/2(Ppv)  "Ppv (kW)"
  Mux/1 -> Scope 1/1
  [uc] -> Scope 1/2  "uc"
  Subsystem12/1(n_mppt) -> Ppv (kW)18/1
  [Pactiva] -> Subsystem14/1(PkW)
  [uc] -> Subsystem3/1(uc)
  Gain2/1 -> Mux1/1
  Subsystem14/1(wh) -> Ppv (kW)14/1
  Product/1 -> Gain/1
  Mux1/1 -> Scope 1/3
  [Imppt] -> Mux/1  "Imppt (A)"
  Gain/1 -> Saturation1/1
  Subsystem6/2(i_avg) -> Ppv (kW)19/1
  Pmppt 1.3 Seg/1 -> Subsystem12/1(Pmpp)  "Pmppt (kW)"
  [vpv] -> Product/2  "vpv"
  [id] -> Subsystem6/1(Id)
  Saturation1/1 -> [Ppv], Ppv (kW)/1
  [G] -> Gain2/1
  Subsystem14/2(Pw_avg) -> Ppv (kW)22/1
  Subsystem6/1(Ah) -> Ppv (kW)12/1
  [ipv] -> single2double12/1, Product/1  "ipv"
  single2double12/1 -> Mux/2

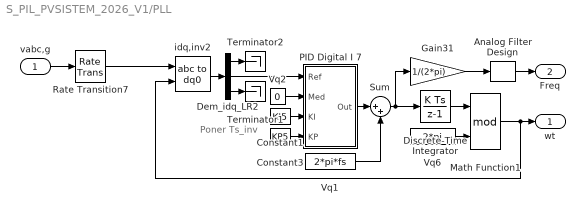
== system S_PIL_PVSISTEM_2026_V1/PLL ==
  note: Poner Ts_inv
  vabc,g : Inport
  Analog Filter Design : dsparch4/Analog Filter Design  method=Butterworth  filttype=Lowpass  N=8  Wlo=4000  Whi=80  Rp=2  Rs=40
  Constant1 : Constant  Value=KI5  SampleTime=Ts_inv
  Constant3 : Constant  Value=KP5  SampleTime=Ts_inv
  Dem_idq_LR2 : Demux  Outputs=3
  Discrete-Time Integrator : DiscreteIntegrator  InitialConditionSetting=State (most efficient)  SampleTime=Ts_inv  ICPrevOutput=DiscIntNeverNeededParam  ICPrevScaledInput=DiscIntNeverNeededParam
  Gain31 : Gain  Gain=1/(2*pi)  OutMin=[0.1]
  Math Function1 : Math  Operator=mod  SaturateOnIntegerOverflow=on
  PID Digital I 7 : MATLAB Function  TreatAsAtomicUnit=on
  Rate Transition7 : RateTransition  OutPortSampleTime=Ts_inv
  Sum : Sum  Inputs=|++
  Terminator1 : Terminator
  Terminator2 : Terminator
  Vq1 : Constant  Value=2*pi*fs  SampleTime=Ts_inv
  Vq2 : Constant  Value=0
  Vq6 : Constant  Value=2*pi  SampleTime=Ts_inv
  idq,inv2 : powerlib_meascontrol/Transformations/abc to dq0  Alignment=90 degrees behind phase A axis
  wt : Outport
  Freq : Outport  Port=2
  wires:
  Gain31/1 -> Analog Filter Design/1
  vabc,g/1 -> Rate Transition7/1
  idq,inv2/1 -> Dem_idq_LR2/1
  Vq6/1 -> Math Function1/2
  Discrete-Time Integrator/1 -> Math Function1/1
  Math Function1/1 -> wt/1, idq,inv2/2
  Vq2/1 -> PID Digital I 7/2(Med)
  Dem_idq_LR2/2 -> PID Digital I 7/1(Ref)
  Sum/1 -> Gain31/1, Discrete-Time Integrator/1
  Vq1/1 -> Sum/2
  PID Digital I 7/1(Out) -> Sum/1
  Constant1/1 -> PID Digital I 7/3(KI)
  Constant3/1 -> PID Digital I 7/4(KP)
  Dem_idq_LR2/3 -> Terminator1/1
  Dem_idq_LR2/1 -> Terminator2/1
  Rate Transition7/1 -> idq,inv2/1
  Analog Filter Design/1 -> Freq/1

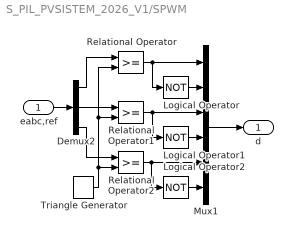
== system S_PIL_PVSISTEM_2026_V1/SPWM ==
  eabc,ref : Inport
  Demux2 : Demux  Outputs=3
  Logical Operator : Logic  Operator=NOT  AllPortsSameDT=off  OutDataTypeStr=boolean
  Logical Operator1 : Logic  Operator=NOT  AllPortsSameDT=off  OutDataTypeStr=boolean
  Logical Operator2 : Logic  Operator=NOT  AllPortsSameDT=off  OutDataTypeStr=boolean
  Mux1 : Mux  Inputs=6
  Relational Operator : RelationalOperator  OutDataTypeStr=boolean  RndMeth=Simplest
  Relational Operator1 : RelationalOperator  OutDataTypeStr=boolean  RndMeth=Simplest
  Relational Operator2 : RelationalOperator  OutDataTypeStr=boolean  RndMeth=Simplest
  Triangle Generator : powerlib_meascontrol/Pulse & Signal Generators/Triangle Generator  Freq=Fc  Phase=0  Ts=Ts_inv
  d : Outport
  wires:
  Logical Operator/1 -> Mux1/2
  Demux2/1 -> Relational Operator/1
  Demux2/2 -> Relational Operator1/1
  Logical Operator1/1 -> Mux1/4
  Relational Operator2/1 -> Mux1/5, Logical Operator2/1
  Triangle Generator/1 -> Relational Operator2/2, Relational Operator1/2, Relational Operator/2
  Mux1/1 -> d/1
  Relational Operator/1 -> Logical Operator/1, Mux1/1
  Logical Operator2/1 -> Mux1/6
  Demux2/3 -> Relational Operator2/1
  Relational Operator1/1 -> Logical Operator1/1, Mux1/3
  eabc,ref/1 -> Demux2/1

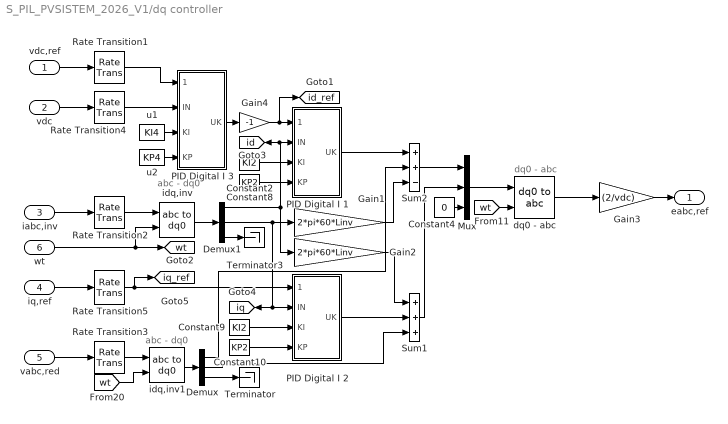
== system S_PIL_PVSISTEM_2026_V1/dq controller ==
  note: dq0 - abc
  note: abc - dq0
  note: abc - dq0
  vdc,ref : Inport
  vdc : Inport  Port=2
  iabc,inv : Inport  Port=3
  iq,ref : Inport  Port=4
  vabc,red : Inport  Port=5
  wt : Inport  Port=6
  Constant10 : Constant  Value=KP2  SampleTime=Ts4
  Constant2 : Constant  Value=KI2  SampleTime=Ts4
  Constant4 : Constant  Value=0  SampleTime=Ts4
  Constant8 : Constant  Value=KP2  SampleTime=Ts4
  Constant9 : Constant  Value=KI2  SampleTime=Ts4
  Demux : Demux  Outputs=3
  Demux1 : Demux  Outputs=3
  Gain1 : Gain  Gain=2*pi*60*Linv
  Gain2 : Gain  Gain=2*pi*60*Linv
  Gain3 : Gain  Gain=(2/vdc)
  Gain4 : Gain  Gain=-1
  Mux : Mux  Inputs=3
  PID Digital I 1 : MATLAB Function  TreatAsAtomicUnit=on
  PID Digital I 2 : MATLAB Function  TreatAsAtomicUnit=on
  PID Digital I 3 : MATLAB Function  TreatAsAtomicUnit=on
  Rate Transition{1..5} (5 alike) : RateTransition  OutPortSampleTime=Ts4
  Sum1 : Sum  Inputs=+++
  Sum2 : Sum  Inputs=++-
  Terminator : Terminator
  Terminator3 : Terminator
  dq0 - abc : powerlib_meascontrol/Transformations/dq0 to abc  Alignment=90 degrees behind phase A axis
  idq,inv : powerlib_meascontrol/Transformations/abc to dq0  Alignment=90 degrees behind phase A axis
  idq,inv1 : powerlib_meascontrol/Transformations/abc to dq0  Alignment=90 degrees behind phase A axis
  u1 : Constant  Value=KI4  SampleTime=Ts4
  u2 : Constant  Value=KP4  SampleTime=Ts4
  eabc,ref : Outport
  tag scope: id=global, id_ref=global, iq=global, iq_ref=global, wt=global
  wires:
  vabc,red/1 -> Rate Transition3/1
  Rate Transition4/1 -> PID Digital I 3/2(IN)
  Demux/2 -> Sum1/3
  Demux1/2 -> PID Digital I 2/2(IN), [iq], Gain1/1
  PID Digital I 1/1(UK) -> Sum2/1
  Gain4/1 -> [id_ref], PID Digital I 1/1(IN_ref)
  Sum1/1 -> Mux/2
  Mux/1 -> dq0 - abc/1
  Constant4/1 -> Mux/3
  [wt] -> dq0 - abc/2
  Demux/3 -> Terminator/1
  Demux1/1 -> [id], PID Digital I 1/2(IN), Gain2/1
  Constant8/1 -> PID Digital I 1/4(KP)
  Rate Transition5/1 -> [iq_ref], PID Digital I 2/1(IN_ref)
  idq,inv1/1 -> Demux/1
  iq,ref/1 -> Rate Transition5/1
  idq,inv/1 -> Demux1/1
  Constant9/1 -> PID Digital I 2/3(KI)
  u1/1 -> PID Digital I 3/3(KI)
  vdc,ref/1 -> Rate Transition1/1
  Constant10/1 -> PID Digital I 2/4(KP)
  vdc/1 -> Rate Transition4/1
  Constant2/1 -> PID Digital I 1/3(KI)
  iabc,inv/1 -> Rate Transition2/1
  Rate Transition2/1 -> idq,inv/1
  Demux1/3 -> Terminator3/1
  Rate Transition3/1 -> idq,inv1/1
  u2/1 -> PID Digital I 3/4(KP)
  PID Digital I 2/1(UK) -> Sum1/2
  Sum2/1 -> Mux/1
  Demux/1 -> Sum2/2
  Gain2/1 -> Sum1/1
  Gain1/1 -> Sum2/3
  [wt] -> idq,inv1/2
  wt/1 -> [wt], idq,inv/2
  dq0 - abc/1 -> Gain3/1
  PID Digital I 3/1(UK) -> Gain4/1
  Rate Transition1/1 -> PID Digital I 3/1(IN_ref)
  Gain3/1 -> eabc,ref/1

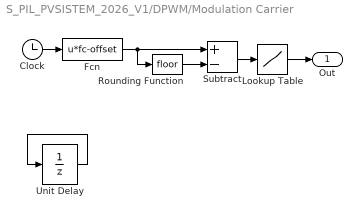
== system S_PIL_PVSISTEM_2026_V1/DPWM/Modulation Carrier ==
  Clock : Clock
  Fcn : Fcn  Expr=u*fc-offset
  Lookup Table : Lookup  InputValues=[0 .5 1]  Table=[range(1) range(2) range(1)]  LookUpMeth=Interpolation-Use End Values
  Rounding Function : Rounding
  Subtract : Sum  Inputs=+-
  Unit Delay : UnitDelay  SampleTime=si
  Out : Outport
  wires:
  Lookup Table/1 -> Out/1
  Subtract/1 -> Lookup Table/1
  Rounding Function/1 -> Subtract/2
  Fcn/1 -> Rounding Function/1, Subtract/1
  Clock/1 -> Fcn/1
  Unit Delay/1 -> Unit Delay/1

== system S_PIL_PVSISTEM_2026_V1/Measurements 1/Subsystem ==
  I : Inport
  Clock : Clock
  Constant : Constant  Value=0.1
  MATLAB Function : MATLAB Function  TreatAsAtomicUnit=on
  O : Outport
  wires:
  MATLAB Function/1(y) -> O/1
  I/1 -> MATLAB Function/1(u)
  Constant/1 -> MATLAB Function/3(t_on)
  Clock/1 -> MATLAB Function/2(time)

== system S_PIL_PVSISTEM_2026_V1/Measurements 2/Subsystem12 ==
  Pmpp : Inport
  Ppv : Inport  Port=2
  Clock : Clock
  Constant : Constant  Value=0.1
  Constant1 : Constant  Value=1.3
  MATLAB Function : MATLAB Function  TreatAsAtomicUnit=on
  n_mppt : Outport
  wires:
  MATLAB Function/1(efficiency) -> n_mppt/1
  Constant/1 -> MATLAB Function/4(t_start)
  Constant1/1 -> MATLAB Function/5(t_end)
  Pmpp/1 -> MATLAB Function/1(Pmpp)
  Ppv/1 -> MATLAB Function/2(Pactual)
  Clock/1 -> MATLAB Function/3(time)

== system S_PIL_PVSISTEM_2026_V1/Measurements 2/Subsystem14 ==
  PkW : Inport
  Clock : Clock
  Constant : Constant  Value=0.1
  Constant1 : Constant  Value=1.3
  MATLAB Function : MATLAB Function  TreatAsAtomicUnit=on
  wh : Outport
  Pw_avg : Outport  Port=2
  wires:
  MATLAB Function/1(energy_wh) -> wh/1
  PkW/1 -> MATLAB Function/1(power_kw)
  Clock/1 -> MATLAB Function/2(time)
  Constant/1 -> MATLAB Function/3(t_start)
  Constant1/1 -> MATLAB Function/4(t_end)
  MATLAB Function/2(power_avg) -> Pw_avg/1

== system S_PIL_PVSISTEM_2026_V1/Measurements 2/Subsystem3 ==
  uc : Inport
  Clock : Clock
  Constant : Constant  Value=0.1
  Constant1 : Constant  Value=1.3
  MATLAB Function : MATLAB Function  TreatAsAtomicUnit=on
  uc_avg : Outport
  wires:
  MATLAB Function/1(uc_avg) -> uc_avg/1
  Constant/1 -> MATLAB Function/3(t_start)
  Constant1/1 -> MATLAB Function/4(t_end)
  uc/1 -> MATLAB Function/1(uc)
  Clock/1 -> MATLAB Function/2(time)

== system S_PIL_PVSISTEM_2026_V1/Measurements 2/Subsystem6 ==
  Id : Inport
  Clock : Clock
  Constant : Constant  Value=0.1
  Constant1 : Constant  Value=1.3
  MATLAB Function : MATLAB Function  TreatAsAtomicUnit=on
  Ah : Outport
  i_avg : Outport  Port=2
  wires:
  MATLAB Function/1(ah) -> Ah/1
  Id/1 -> MATLAB Function/1(current)
  Clock/1 -> MATLAB Function/2(time)
  Constant/1 -> MATLAB Function/3(t_start)
  Constant1/1 -> MATLAB Function/4(t_end)
  MATLAB Function/2(i_avg) -> i_avg/1

== matlab function S_PIL_PVSISTEM_2026_V1/Measurements 2/Look-Up Table-Based MPPT (LTB MPPT) ==
  data: G input; i_mpp output; dIL input
function i_mpp = fcn(G, dIL)
% MPP current reference generation using a G-to-Impp lookup table.
%
% G       : irradiance input
% dIL     : peak-to-peak inductor-current ripple compensation
%
% Output:
% i_mpp   : compensated MPP current reference
%
% The lookup table covers G = 50...1200 W/m^2 with a 10 W/m^2 step.
% Linear interpolation is used within the table and extrapolation is
% applied outside the tabulated irradiance range.

persistent G_tab Impp_tab

if isempty(G_tab)

    G_tab = single(50:10:1200);

    Impp_tab = coder.const(double([ ...
    0.79 0.95 1.10 1.26 1.42 1.58 1.74 1.89 2.05 2.21 ...
    2.36 2.53 2.68 2.84 3.00 3.15 3.31 3.47 3.63 3.78 ...
    3.95 4.10 4.26 4.41 4.58 4.73 4.89 5.05 5.21 5.36 ...
    5.52 5.68 5.84 5.99 6.15 6.31 6.46 6.62 6.78 6.94 ...
    7.09 7.25 7.41 7.57 7.72 7.88 8.04 8.20 8.36 8.51 ...
    8.67 8.83 8.98 9.13 9.29 9.45 9.61 9.76 9.92 10.08 ...
    10.24 10.39 10.55 10.71 10.86 11.02 11.18 11.33 11.49 11.64 ...
    11.80 11.96 12.11 12.28 12.44 12.60 12.75 12.90 13.06 13.21 ...
    13.37 13.52 13.68 13.85 14.01 14.16 14.31 14.47 14.62 14.77 ...
    14.92 15.10 15.25 15.41 15.56 15.71 15.86 16.04 16.19 16.34 ...
    16.49 16.64 16.80 16.96 17.12 17.27 17.42 17.57 17.75 17.90 ...
    18.05 18.20 18.35 18.53 18.68 18.83
    ]));

end

% Nominal MPP-current interpolation
I_mpp_nom = interp1(G_tab, Impp_tab, G, 'linear', 'extrap');

% Inductor-current ripple compensation
i_mpp = I_mpp_nom - (dIL/2)*1.1;


% Prevent negative current-reference values
i_mpp = max(i_mpp, 0);

end

== matlab function S_PIL_PVSISTEM_2026_V1/dq controller/PID Digital I 1 ==
  data: IN_ref input; UK output; IN input; KI input; KP input
function UK = fcn(IN_ref, IN, KI, KP)

 %Initial values
 persistent  ek uk
 persistent  ek_1 uk_1
 if isempty(ek)
    ek =0;
    uk =0;
    ek_1 =0;
    uk_1 =0;
 end
ek=IN_ref-IN;
uk=ek*(KP+KI)-ek_1*KP+uk_1;
if(uk>1000)
    uk=1000;
end
if(uk<-1000)
    uk=-1000;
end
ek_1=ek;
uk_1=uk;
UK=uk;
end

== matlab function S_PIL_PVSISTEM_2026_V1/dq controller/PID Digital I 2 ==
  data: IN_ref input; UK output; IN input; KI input; KP input
function UK = fcn(IN_ref, IN, KI, KP)

 %Initial values
 persistent  ek uk
 persistent  ek_1 uk_1
 if isempty(ek)
    ek =0;
    uk =0;
    ek_1 =0;
    uk_1 =0;
 end
ek=IN_ref-IN;
uk=ek*(KP+KI)-ek_1*KP+uk_1;
if(uk>1000)
    uk=1000;
end
if(uk<-1000)
    uk=-1000;
end
ek_1=ek;
uk_1=uk;
UK=uk;
end

== matlab function S_PIL_PVSISTEM_2026_V1/dq controller/PID Digital I 3 ==
  data: IN_ref input; UK output; IN input; KI input; KP input
function UK = fcn(IN_ref, IN, KI, KP)

 %Initial values
 persistent  ek uk
 persistent  ek_1 uk_1
 if isempty(ek)
    ek =0;
    uk =0;
    ek_1 =0;
    uk_1 =0;
 end
ek=IN_ref-IN;
uk=ek*(KP+KI)-ek_1*KP+uk_1;
if(uk>60)
    uk=60;
end
if(uk<-60)
    uk=-60;
end
ek_1=ek;
uk_1=uk;
UK=uk;
end

== matlab function S_PIL_PVSISTEM_2026_V1/PLL/PID Digital I 7 ==
  data: Ref input; Out output; Med input; KI input; KP input
function Out = fcn(Ref, Med, KI, KP)

 %Valores iniciales de las conStantes del controlador
 persistent  ek uk
 persistent  ek_1 uk_1
 if isempty(ek)
    ek =0;
    uk =0;
    ek_1 =0;
    uk_1 =0;
 end
ek=Ref-Med;
%uk=ek*(KP+KI)-ek_1*KP+uk_1;
uk=KP*ek+KI*ek+KI*ek_1;
ek_1=ek;
uk_1=uk;
Out=uk;
end

== matlab function S_PIL_PVSISTEM_2026_V1/Cont Real Est1/Look-Up Table-Based MPPT ==
  data: G input; i_mpp output; dIL input
function i_mpp = fcn(G, dIL)
% MPP current reference generation using a G-to-Impp lookup table.
%
% G       : irradiance input
% dIL     : peak-to-peak inductor-current ripple compensation
%
% Output:
% i_mpp   : compensated MPP current reference
%
% The lookup table covers G = 50...1200 W/m^2 with a 10 W/m^2 step.
% Linear interpolation is used within the table and extrapolation is
% applied outside the tabulated irradiance range.

persistent G_tab Impp_tab

if isempty(G_tab)

    G_tab = single(50:10:1200);

    Impp_tab = coder.const(double([ ...
    0.79 0.95 1.10 1.26 1.42 1.58 1.74 1.89 2.05 2.21 ...
    2.36 2.53 2.68 2.84 3.00 3.15 3.31 3.47 3.63 3.78 ...
    3.95 4.10 4.26 4.41 4.58 4.73 4.89 5.05 5.21 5.36 ...
    5.52 5.68 5.84 5.99 6.15 6.31 6.46 6.62 6.78 6.94 ...
    7.09 7.25 7.41 7.57 7.72 7.88 8.04 8.20 8.36 8.51 ...
    8.67 8.83 8.98 9.13 9.29 9.45 9.61 9.76 9.92 10.08 ...
    10.24 10.39 10.55 10.71 10.86 11.02 11.18 11.33 11.49 11.64 ...
    11.80 11.96 12.11 12.28 12.44 12.60 12.75 12.90 13.06 13.21 ...
    13.37 13.52 13.68 13.85 14.01 14.16 14.31 14.47 14.62 14.77 ...
    14.92 15.10 15.25 15.41 15.56 15.71 15.86 16.04 16.19 16.34 ...
    16.49 16.64 16.80 16.96 17.12 17.27 17.42 17.57 17.75 17.90 ...
    18.05 18.20 18.35 18.53 18.68 18.83
    ]));

end

% Nominal MPP-current interpolation
I_mpp_nom = interp1(G_tab, Impp_tab, G, 'linear', 'extrap');

% Inductor-current ripple compensation
i_mpp = I_mpp_nom - dIL;

% Prevent negative current-reference values
i_mpp = max(i_mpp, 0);

end

== matlab function S_PIL_PVSISTEM_2026_V1/Cont Real Est2/EHGO using Eq. (13) ==
  data: y_k input; alpha_1 input; alpha_2 input; epsilon input; Kdpwm input; vdc input; L input; Ts input; u_c_k input; z_hat_k input; z_hat_next output
function z_hat_next = fcn(y_k, alpha_1, alpha_2, epsilon, ...
                          Kdpwm, vdc, L, Ts, u_c_k, z_hat_k)
% Discrete-time extended high-gain observer (EHGO) used in the
% FL-EHGO structure with proportional auxiliary control.
%
% Inputs:
%   y_k        : measured output y[k] = i_pv[k]
%   alpha_1    : first EHGO coefficient
%   alpha_2    : second EHGO coefficient
%   epsilon    : EHGO tuning parameter
%   Kdpwm      : digital PWM gain
%   vdc        : dc-bus voltage
%   L          : boost-converter inductance
%   Ts         : sampling period
%   u_c_k      : converter control input u_c[k]
%   z_hat_k    : EHGO estimates [z_hat[k]; sigma_hat[k]]
%
% Output:
%   z_hat_next : EHGO estimates at k+1

z_hat_next = zeros(2,1);

% Observer estimation error
e_obs_k = y_k - z_hat_k(1);

% EHGO update according to Eq. (13)
% The nominal term b_hat is neglected in the practical implementation.

z_hat_next(1) = z_hat_k(1) + Ts * ( ...
    z_hat_k(2) + ...
    ((Kdpwm/L)*vdc)*u_c_k + ...
    (alpha_1/(epsilon*Ts))*e_obs_k );

z_hat_next(2) = z_hat_k(2) + Ts * ( ...
    (alpha_2/(epsilon^2*Ts^2))*e_obs_k );

end

== matlab function S_PIL_PVSISTEM_2026_V1/Measurements 1/Subsystem/MATLAB Function ==
  data: y output; u input; time input; t_on input
function y = time_gate(u, time, t_on)
%#codegen
% Si time < t_on => y = 0
% Si time >= t_on => y = u
%
% Entradas:
%   u     : señal de entrada (esc. o vector)
%   time  : tiempo actual (s)
%   t_on  : tiempo umbral para habilitar (s)
%
% Salida:
%   y     : señal gated

if time < t_on
    y = zeros(size(u), 'like', u);  % mantiene tipo/dimensión de u
else
    y = u;
end
end
